simulink model "SlidingMode_uitwerking"  (Simulink 7.5)
settings: Solver=ode45  StartTime=0.0  StopTime=Tsim  RelTol=1e-3
undefined symbols (not defined in the file or in its folder): delta, xInit
settings Model: Creator=DRijlaars  LastModifiedBy=s050760
settings OptimizationCC: InitFltsAndDblsToZero=on
settings DebuggingCC: StrictBusMsg=Warning

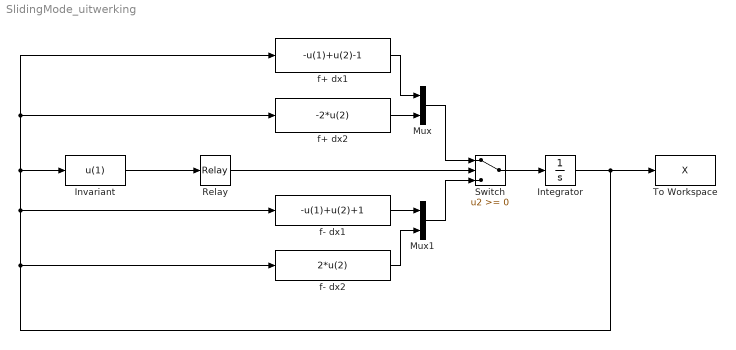
== system SlidingMode_uitwerking ==
  Integrator : Integrator  InitialCondition=xInit
  Invariant : Fcn  Expr=u(1)
  Mux : Mux  Inputs=2
  Mux1 : Mux  Inputs=2
  Relay : Relay  OnSwitchValue=delta  OffSwitchValue=-delta  OnOutputValue=0.01  OffOutputValue=-0.01  OutDataType=sfix(16)  OutScaling=2^0
  Switch : Switch  OutDataType=sfix(16)  OutScaling=2^0
  To Workspace : ToWorkspace  VariableName=X  SampleTime=-1  SaveFormat=Structure With Time
  f+ dx1 : Fcn  Expr=-u(1)+u(2)-1
  f+ dx2 : Fcn  Expr=-2*u(2)
  f- dx1 : Fcn  Expr=-u(1)+u(2)+1
  f- dx2 : Fcn  Expr=2*u(2)
  wires:
  Integrator/1 -> To Workspace/1, f- dx2/1, Invariant/1, f+ dx1/1, f+ dx2/1, f- dx1/1
  Switch/1 -> Integrator/1
  Invariant/1 -> Relay/1
  Mux/1 -> Switch/1
  Mux1/1 -> Switch/3
  f- dx1/1 -> Mux1/1
  f- dx2/1 -> Mux1/2
  f+ dx2/1 -> Mux/2
  f+ dx1/1 -> Mux/1
  Relay/1 -> Switch/2
